simulink model "Case1_Sim"  (R2020b)
settings: Solver=FixedStepAuto  StartTime=0.0  StopTime=0.8  FixedStep=Ts  RelTol=1e-3
values from neighbouring files (symbols this model uses):
  m = 5/100    (= 0.05)    [Case1_SimPara.m]
  Sbase = 1    [Case1_SimPara.m]
  Ts = 1/Fs    (= 0.0001)    [Case1_SimPara.m]
  Vbase = 1    [Case1_SimPara.m]
  w_droop = 10*2*pi    (= 62.8318530718)    [Case1_SimPara.m]
  w_pll = 10*2*pi    (= 62.8318530718)    [Case1_SimPara.m]
  w_tau = 1e3*2*pi    (= 6283.18530718)    [Case1_SimPara.m]
  Wbase = 2*pi*50    (= 314.159265359)    [Case1_SimPara.m]
undefined symbols (not defined in the file or in its folder): DiscIntNeverNeededParam
libraries: SimplexPS x22, powerlib x1
(part 2 of 2)

== system Case1_Sim/PLL (vabc -> vq)5 ==
  note: Gpll
  note: Measurement
  vabc : Inport
  Atan2 : Trigonometry  Operator=atan2
  Constant1 : Constant
  Constant2 : Constant  Value=theta0
  Constant3 : Constant
  Constant4 : Constant  Value=2*pi
  Constant5 : Constant  Commented=on  Value=pi/2/2
  Constant6 : Constant  Value=0
  Constant7 : Constant  Commented=on  Value=2*pi
  Demux1 : Demux  Outputs=2
  Discrete PI : SimplexPS/Discrete PI  Kp=w_pll  Ki=w_pll*w_pll/4  xmax=inf  xmin=-inf  Ts=Ts
      settings: SourceProductName=Simplex Power Systems
  Discrete-Time Integrator : DiscreteIntegrator  SampleTime=Ts  ICPrevOutput=DiscIntNeverNeededParam  ICPrevScaledInput=DiscIntNeverNeededParam
  Filter p : DiscreteTransferFcn  Commented=on  Numerator=w_tau*Ts  Denominator=[1 ((w_tau*Ts)-1)]  SampleTime=Ts
  From7 : From  Commented=on  GotoTag=theta_PLL_1
  From8 : From  Commented=on  GotoTag=thetag_PLL
  Gain1 : Gain  Gain=Wbase
  Gain2 : Gain  Gain=1/Vbase
  Gain4 : Gain  Gain=1/Wbase
  Gain5 : Gain  Gain=1/pi
  Goto13 : Goto  Commented=on  GotoTag=dtheta_PLL_1
  Math Function1 : Math  Operator=mod  SignedPower=on  SaturateOnIntegerOverflow=on
  Math Function2 : Math  Commented=on  Operator=mod  SignedPower=on  SaturateOnIntegerOverflow=on
  Mux : Mux  Inputs=2
  Scope : Scope  NumInputPorts=4
  Sum : Sum
  Sum1 : Sum
  Sum2 : Sum  Commented=on  Inputs=+-+
  Sum3 : Sum  Commented=on  Inputs=+-
  "abc -> dq (Power-Invariant)" : SimplexPS/abc -> dq (Power-Invariant)  SystemSampleTime=-1  VariantActivationTime=update diagram  Latency=0  AutoFrameSizeCalculation=off
      settings: SourceProductName=Simplex Power Systems
  w : Outport
  theta : Outport  Port=2
  vdq : Outport  Port=3
  vtheta : Outport  Port=4
  wires:
  Math Function1/1 -> theta/1, [theta], "abc -> dq (Power-Invariant)"/2
  Constant3/1 -> Gain1/1
  Demux1/1 -> [vd]
  [theta] -> Mux/2  "theta"
  Gain5/1 -> Scope/4
  [vd] -> Scope/1  "vd"
  [theta0] -> Mux/1  "theta0"
  [w] -> Gain4/1  "w"
  Gain4/1 -> Scope/3
  Mux/1 -> Gain5/1
  [vq] -> Scope/2  "vq"
  Gain2/1 -> Discrete PI/2
  Constant2/1 -> Sum1/2, [theta0]
  Sum1/1 -> Math Function1/1
  Discrete-Time Integrator/1 -> Sum1/1
  Gain1/1 -> Sum/2
  Sum/1 -> Discrete-Time Integrator/1, w/1, [w]
  Discrete PI/1 -> Sum/1
  Constant1/1 -> Discrete PI/1
  Constant6/1 -> Discrete PI/3, Discrete PI/4
  Demux1/2 -> Gain2/1, [vq]
  Constant4/1 -> Math Function1/2
  "abc -> dq (Power-Invariant)"/1 -> Demux1/1, vdq/1
  vabc/1 -> "abc -> dq (Power-Invariant)"/1
  Atan2/1 -> vtheta/1
  From8/1 -> Sum2/2
  Sum2/1 -> Math Function2/1
  From7/1 -> Sum2/1
  Constant7/1 -> Math Function2/2
  Math Function2/1 -> Sum3/1
  Constant5/1 -> Sum3/2, Sum2/3
  Sum3/1 -> Goto13/1
  [vq] -> Atan2/1
  [vd] -> Atan2/2

== system Case1_Sim/PLL (vabc -> vq)6 ==
  note: Gpll
  note: Measurement
  vabc : Inport
  Atan2 : Trigonometry  Operator=atan2
  Constant1 : Constant
  Constant2 : Constant  Value=theta0
  Constant3 : Constant
  Constant4 : Constant  Value=2*pi
  Constant5 : Constant  Commented=on  Value=pi/2/2
  Constant6 : Constant  Value=0
  Constant7 : Constant  Commented=on  Value=2*pi
  Demux1 : Demux  Outputs=2
  Discrete PI : SimplexPS/Discrete PI  Kp=w_pll  Ki=w_pll*w_pll/4  xmax=inf  xmin=-inf  Ts=Ts
      settings: SourceProductName=Simplex Power Systems
  Discrete-Time Integrator : DiscreteIntegrator  SampleTime=Ts  ICPrevOutput=DiscIntNeverNeededParam  ICPrevScaledInput=DiscIntNeverNeededParam
  Filter p : DiscreteTransferFcn  Commented=on  Numerator=w_tau*Ts  Denominator=[1 ((w_tau*Ts)-1)]  SampleTime=Ts
  From7 : From  Commented=on  GotoTag=theta_PLL_1
  From8 : From  Commented=on  GotoTag=thetag_PLL
  Gain1 : Gain  Gain=Wbase
  Gain2 : Gain  Gain=1/Vbase
  Gain4 : Gain  Gain=1/Wbase
  Gain5 : Gain  Gain=1/pi
  Goto13 : Goto  Commented=on  GotoTag=dtheta_PLL_1
  Math Function1 : Math  Operator=mod  SignedPower=on  SaturateOnIntegerOverflow=on
  Math Function2 : Math  Commented=on  Operator=mod  SignedPower=on  SaturateOnIntegerOverflow=on
  Mux : Mux  Inputs=2
  Scope : Scope  NumInputPorts=4
  Sum : Sum
  Sum1 : Sum
  Sum2 : Sum  Commented=on  Inputs=+-+
  Sum3 : Sum  Commented=on  Inputs=+-
  "abc -> dq (Power-Invariant)" : SimplexPS/abc -> dq (Power-Invariant)  SystemSampleTime=-1  VariantActivationTime=update diagram  Latency=0  AutoFrameSizeCalculation=off
      settings: SourceProductName=Simplex Power Systems
  w : Outport
  theta : Outport  Port=2
  vdq : Outport  Port=3
  vtheta : Outport  Port=4
  wires:
  Math Function1/1 -> theta/1, [theta], "abc -> dq (Power-Invariant)"/2
  Constant3/1 -> Gain1/1
  Demux1/1 -> [vd]
  [theta] -> Mux/2  "theta"
  Gain5/1 -> Scope/4
  [vd] -> Scope/1  "vd"
  [theta0] -> Mux/1  "theta0"
  [w] -> Gain4/1  "w"
  Gain4/1 -> Scope/3
  Mux/1 -> Gain5/1
  [vq] -> Scope/2  "vq"
  Gain2/1 -> Discrete PI/2
  Constant2/1 -> Sum1/2, [theta0]
  Sum1/1 -> Math Function1/1
  Discrete-Time Integrator/1 -> Sum1/1
  Gain1/1 -> Sum/2
  Sum/1 -> Discrete-Time Integrator/1, w/1, [w]
  Discrete PI/1 -> Sum/1
  Constant1/1 -> Discrete PI/1
  Constant6/1 -> Discrete PI/3, Discrete PI/4
  Demux1/2 -> Gain2/1, [vq]
  Constant4/1 -> Math Function1/2
  "abc -> dq (Power-Invariant)"/1 -> Demux1/1, vdq/1
  vabc/1 -> "abc -> dq (Power-Invariant)"/1
  Atan2/1 -> vtheta/1
  From8/1 -> Sum2/2
  Sum2/1 -> Math Function2/1
  From7/1 -> Sum2/1
  Constant7/1 -> Math Function2/2
  Math Function2/1 -> Sum3/1
  Constant5/1 -> Sum3/2, Sum2/3
  Sum3/1 -> Goto13/1
  [vq] -> Atan2/1
  [vd] -> Atan2/2

== system Case1_Sim/PLL (vabc -> vq)7 ==
  note: Gpll
  note: Measurement
  vabc : Inport
  Atan2 : Trigonometry  Operator=atan2
  Constant1 : Constant
  Constant2 : Constant  Value=theta0
  Constant3 : Constant
  Constant4 : Constant  Value=2*pi
  Constant5 : Constant  Commented=on  Value=pi/2/2
  Constant6 : Constant  Value=0
  Constant7 : Constant  Commented=on  Value=2*pi
  Demux1 : Demux  Outputs=2
  Discrete PI : SimplexPS/Discrete PI  Kp=w_pll  Ki=w_pll*w_pll/4  xmax=inf  xmin=-inf  Ts=Ts
      settings: SourceProductName=Simplex Power Systems
  Discrete-Time Integrator : DiscreteIntegrator  SampleTime=Ts  ICPrevOutput=DiscIntNeverNeededParam  ICPrevScaledInput=DiscIntNeverNeededParam
  Filter p : DiscreteTransferFcn  Commented=on  Numerator=w_tau*Ts  Denominator=[1 ((w_tau*Ts)-1)]  SampleTime=Ts
  From7 : From  Commented=on  GotoTag=theta_PLL_1
  From8 : From  Commented=on  GotoTag=thetag_PLL
  Gain1 : Gain  Gain=Wbase
  Gain2 : Gain  Gain=1/Vbase
  Gain4 : Gain  Gain=1/Wbase
  Gain5 : Gain  Gain=1/pi
  Goto13 : Goto  Commented=on  GotoTag=dtheta_PLL_1
  Math Function1 : Math  Operator=mod  SignedPower=on  SaturateOnIntegerOverflow=on
  Math Function2 : Math  Commented=on  Operator=mod  SignedPower=on  SaturateOnIntegerOverflow=on
  Mux : Mux  Inputs=2
  Scope : Scope  NumInputPorts=4
  Sum : Sum
  Sum1 : Sum
  Sum2 : Sum  Commented=on  Inputs=+-+
  Sum3 : Sum  Commented=on  Inputs=+-
  "abc -> dq (Power-Invariant)" : SimplexPS/abc -> dq (Power-Invariant)  SystemSampleTime=-1  VariantActivationTime=update diagram  Latency=0  AutoFrameSizeCalculation=off
      settings: SourceProductName=Simplex Power Systems
  w : Outport
  theta : Outport  Port=2
  vdq : Outport  Port=3
  vtheta : Outport  Port=4
  wires:
  Math Function1/1 -> theta/1, [theta], "abc -> dq (Power-Invariant)"/2
  Constant3/1 -> Gain1/1
  Demux1/1 -> [vd]
  [theta] -> Mux/2  "theta"
  Gain5/1 -> Scope/4
  [vd] -> Scope/1  "vd"
  [theta0] -> Mux/1  "theta0"
  [w] -> Gain4/1  "w"
  Gain4/1 -> Scope/3
  Mux/1 -> Gain5/1
  [vq] -> Scope/2  "vq"
  Gain2/1 -> Discrete PI/2
  Constant2/1 -> Sum1/2, [theta0]
  Sum1/1 -> Math Function1/1
  Discrete-Time Integrator/1 -> Sum1/1
  Gain1/1 -> Sum/2
  Sum/1 -> Discrete-Time Integrator/1, w/1, [w]
  Discrete PI/1 -> Sum/1
  Constant1/1 -> Discrete PI/1
  Constant6/1 -> Discrete PI/3, Discrete PI/4
  Demux1/2 -> Gain2/1, [vq]
  Constant4/1 -> Math Function1/2
  "abc -> dq (Power-Invariant)"/1 -> Demux1/1, vdq/1
  vabc/1 -> "abc -> dq (Power-Invariant)"/1
  Atan2/1 -> vtheta/1
  From8/1 -> Sum2/2
  Sum2/1 -> Math Function2/1
  From7/1 -> Sum2/1
  Constant7/1 -> Math Function2/2
  Math Function2/1 -> Sum3/1
  Constant5/1 -> Sum3/2, Sum2/3
  Sum3/1 -> Goto13/1
  [vd] -> Atan2/2
  [vq] -> Atan2/1
